simulink model "alignmentdoc"  (Simulink 5.0)
settings: Solver=ode45  StartTime=0.0  StopTime=20  RelTol=1e-3
undefined symbols (not defined in the file or in its folder): gfprimfd, slcm
libraries: dspsigops x2, commblkcod2 x2, dspsnks4 x2, commrandsrc2 x1, commsink2 x1
settings Model: CovMetricSettings=d  Creator=ptrow  LastModifiedBy=agaltman  SaveTime=off  SaveOutput=off  SignalLoggingName=logsOut  BlockReductionOpt=off  BooleanDataType=off  ZeroCrossControl=UseLocalSettings  RTWMathFcnLibMatFile=iso_c_tmw.mat  RTWOptions=-aRollThreshold=5

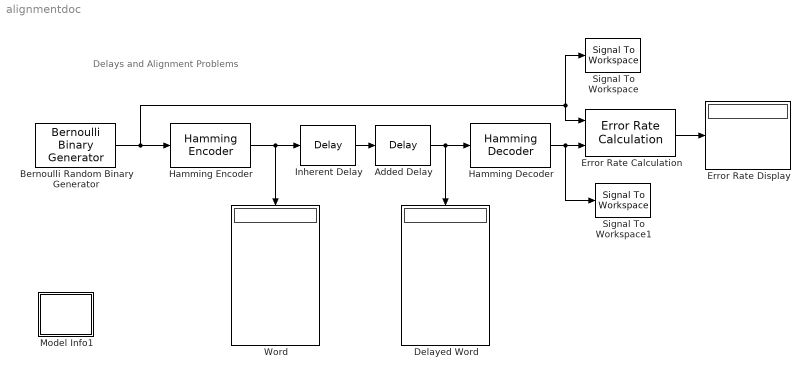
== system alignmentdoc ==
  note: Delays and Alignment Problems
  Added Delay : dspsigops/Delay  dly_unit=Samples  delay=0  ic_detail=off  dif_ic_for_ch=off  dif_ic_for_dly=off  ic=0  reset_popup=None
  Bernoulli Random Binary Generator : commrandsrc2/Bernoulli Binary Generator  P=0.5  seed=89  Ts=1  frameBased=on  sampPerFrame=4  orient=off
  Delayed Word : Display
      settings: Orientation=down
  Error Rate Calculation : commsink2/Error Rate Calculation  N=0  st_delay=0  cp_mode=Entire frame  subframe=[]  PMode=Port  WsName=ErrorVec  RsMode2=off  stop=off  numErr=100  maxBits=1e5
  Error Rate Display : Display
  Hamming Decoder : commblkcod2/Hamming Decoder  n=7  k=gfprimfd(3,'min')
  Hamming Encoder : commblkcod2/Hamming Encoder  n=7  k=gfprimfd(3,'min')
  Inherent Delay : dspsigops/Delay  dly_unit=Samples  delay=1  ic_detail=off  dif_ic_for_ch=off  dif_ic_for_dly=off  ic=0  reset_popup=None
  Model Info1 : Subsystem  LoadFcn=slcm LoadBlock;  InitFcn=slcm('UpdateAllCMBlocksInThisModelInit')  mask(CMBlock){InitialSaveTempField=, InitialBlockCM=none, BlockCM=none, Frame=on, SaveTempField=, DisplayStringWithTags=Info, MaskDisplayString=Info, HorizontalTextAlignment=Center, LeftAlignmentValue=0.5, SourceBlockDiagram=alignmentdoc_on_disk_tp422683, TagMaxNumber=20, CMTag1=, CMTag2=, CMTag3=, CMTag4=, CMTag5=, CMTag6=, CMTag7=, CMTag8=, CMTag9=, CMTag10=, CMTag11=, CMTag12=, CMTag13=, CMTag14=, CMTag15=, CMTag16=, CMTag17=, CMTag18=, CMTag19=, CMTag20=}
      mask help: This block allows revision control information to be displayed within the model.
      settings: CopyFcn=slcm CopyBlock;  DeleteFcn=slcm Cancel;  PostSaveFcn=slcm('UpdateAllCMBlocksInThisModel')  NameChangeFcn=slcm Rename;  OpenFcn=commdemohelp;
      mask Display: text(str2num(LeftAlignmentValue), 0.5, MaskDisplayString, 'HorizontalAlignment', HorizontalTextAlignment)
  Signal To Workspace : dspsnks4/Signal To Workspace  VariableName=tx  FrameMode=Concatenate frames (2-D array)
  Signal To Workspace1 : dspsnks4/Signal To Workspace  VariableName=rx  FrameMode=Concatenate frames (2-D array)
  Word : Display
      settings: Orientation=down
  wires:
  Bernoulli Random Binary Generator/1 -> Hamming Encoder/1, Error Rate Calculation/1, Signal To Workspace/1
  Hamming Decoder/1 -> Error Rate Calculation/2, Signal To Workspace1/1
  Hamming Encoder/1 -> Word/1, Inherent Delay/1
  Inherent Delay/1 -> Added Delay/1
  Error Rate Calculation/1 -> Error Rate Display/1
  Added Delay/1 -> Hamming Decoder/1, Delayed Word/1

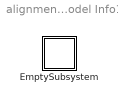
== system alignmentdoc/Model Info1 ==
  EmptySubsystem : Subsystem

== system alignmentdoc/Model Info1/EmptySubsystem ==
